simulink model "six_plus_six_AcmsteeringV09_main_2lfrf"  (R2014a)
settings: Solver=FixedStepDiscrete  StartTime=0.0  StopTime=10.0  FixedStep=0.0005  RelTol=1e-3
InitFcn:
  | Veh_Par_wxt
undefined symbols (not defined in the file or in its folder): acc_spdctl, ag_thr, B, bra_em, bra_pre_gz2, bra_pre_gz34, bra_pre_yd, brakepre_dem_data, brakeTrq_dem_data, bratrq_max, ecucoder_acal, eff_tran, ESP_switch, G, guzhang_lf, guzhang_lm, guzhang_lr, guzhang_rf, guzhang_rm, guzhang_rr, kd1, kd2, ki1, ki2, kp1, kp2, L, myFIS, premax, Radius, RC_switch, s_opt_yi, s_opt_zhuan, s_opt_zhuan_add, s_opt_zhuan_table, spd_map_mot, spd_spdctl, speed_thr_park, TCS_switch, tras_ratio, trq_map_mot, trqmax_yd, trqmax_zx, trqmaxneg, v_gain, v_table, v_thr_park, zhidong_bianmazhi, zhidong_down, zhidong_up, zhidong_youmen, zhuanxiang_bianmazhi, zhuanxiang_down, zhuanxiang_up, zhuanxiang_youmen
libraries: simulink x980, ec5744lib x59, fuzblock x2
(part 10 of 25)

== system six_plus_six_AcmsteeringV09_main_2lfrf/Data_input/MCU1_5/MCU1 ==
  input : Inport
  Enable : EnablePort
  Demux : Demux  Outputs=8
  MCU1_ControlTemp_Ad : Sum
  MCU1_ControlTemp_Convert : DataTypeConversion  OutDataTypeStr=uint32
  MCU1_ControlTemp_F : Gain
  MCU1_ControlTemp_L : simulink/Logic and Bit Operations/Bitwise Operator  logicop=AND  UseBitMask=on  BitMask=255  BitMaskRealWorld=Stored Integer
  MCU1_ControlTemp_O : Constant  Value=-40  OutDataTypeStr=single
  MCU1_ControlTemp_S : ArithShift
  MCU1_ControlTemp_Sub : Subsystem
  MCU1_ControlTemp_sat : Saturate  UpperLimit=215  LowerLimit=-40
  MCU1_ControlTempcv : DataTypeConversion
  MCU1_Idc_Ad : Sum
  MCU1_Idc_Convert : DataTypeConversion  OutDataTypeStr=uint32
  MCU1_Idc_F : Gain  Gain=0.1
  MCU1_Idc_L : simulink/Logic and Bit Operations/Bitwise Operator  logicop=AND  UseBitMask=on  BitMask=65535  BitMaskRealWorld=Stored Integer
  MCU1_Idc_O : Constant  Value=-1600  OutDataTypeStr=single
  MCU1_Idc_S : ArithShift
  MCU1_Idc_Sub : Subsystem
  MCU1_Idc_sat : Saturate  UpperLimit=1600  LowerLimit=-1600
  MCU1_Idccv : DataTypeConversion
  MCU1_Idcinput3_Ad : Sum
  MCU1_Idcinput3_C : Constant  Value=256
  MCU1_Idcinput3_P : Product
  MCU1_MotorTemp_Ad : Sum
  MCU1_MotorTemp_Convert : DataTypeConversion  OutDataTypeStr=uint32
  MCU1_MotorTemp_F : Gain
  MCU1_MotorTemp_L : simulink/Logic and Bit Operations/Bitwise Operator  logicop=AND  UseBitMask=on  BitMask=255  BitMaskRealWorld=Stored Integer
  MCU1_MotorTemp_O : Constant  Value=-40  OutDataTypeStr=single
  MCU1_MotorTemp_S : ArithShift
  MCU1_MotorTemp_Sub : Subsystem
  MCU1_MotorTemp_sat : Saturate  UpperLimit=215  LowerLimit=-40
  MCU1_MotorTempcv : DataTypeConversion
  MCU1_PowerFdk_Ad : Sum
  MCU1_PowerFdk_Convert : DataTypeConversion  OutDataTypeStr=uint32
  MCU1_PowerFdk_F : Gain
  MCU1_PowerFdk_L : simulink/Logic and Bit Operations/Bitwise Operator  logicop=AND  UseBitMask=on  BitMask=65535  BitMaskRealWorld=Stored Integer
  MCU1_PowerFdk_O : Constant  Value=0  OutDataTypeStr=single
  MCU1_PowerFdk_S : ArithShift
  MCU1_PowerFdk_Sub : Subsystem
  MCU1_PowerFdk_sat : Saturate  UpperLimit=65535  LowerLimit=0
  MCU1_PowerFdkcv : DataTypeConversion
  MCU1_PowerFdkinput5_Ad : Sum
  MCU1_PowerFdkinput5_C : Constant  Value=256
  MCU1_PowerFdkinput5_P : Product
  MCU1_Udc_Ad : Sum
  MCU1_Udc_Convert : DataTypeConversion  OutDataTypeStr=uint32
  MCU1_Udc_F : Gain  Gain=0.1
  MCU1_Udc_L : simulink/Logic and Bit Operations/Bitwise Operator  logicop=AND  UseBitMask=on  BitMask=65535  BitMaskRealWorld=Stored Integer
  MCU1_Udc_O : Constant  Value=0  OutDataTypeStr=single
  MCU1_Udc_S : ArithShift
  MCU1_Udc_Sub : Subsystem
  MCU1_Udc_sat : Saturate  UpperLimit=1000  LowerLimit=0
  MCU1_Udccv : DataTypeConversion
  MCU1_Udcinput1_Ad : Sum
  MCU1_Udcinput1_C : Constant  Value=256
  MCU1_Udcinput1_P : Product
  MCU1_ControlTemp_Out : Outport
  MCU1_MotorTemp_Out : Outport  Port=2
  MCU1_PowerFdk_Out : Outport  Port=3
  MCU1_Idc_Out : Outport  Port=4
  MCU1_Udc_Out : Outport  Port=5
  wires:
  MCU1_ControlTemp_F/1 -> MCU1_ControlTemp_Ad/1
  MCU1_ControlTemp_O/1 -> MCU1_ControlTemp_Ad/2
  MCU1_ControlTemp_Ad/1 -> MCU1_ControlTemp_sat/1
  MCU1_ControlTemp_sat/1 -> MCU1_ControlTemp_Out/1
  Demux/8 -> MCU1_ControlTemp_Sub/1(In1)
  MCU1_ControlTemp_Sub/1(Out1) -> MCU1_ControlTemp_Convert/1
  MCU1_ControlTemp_Convert/1 -> MCU1_ControlTemp_L/1
  MCU1_ControlTemp_L/1 -> MCU1_ControlTemp_S/1
  MCU1_ControlTemp_S/1 -> MCU1_ControlTempcv/1
  MCU1_ControlTempcv/1 -> MCU1_ControlTemp_F/1
  MCU1_MotorTemp_F/1 -> MCU1_MotorTemp_Ad/1
  MCU1_MotorTemp_O/1 -> MCU1_MotorTemp_Ad/2
  MCU1_MotorTemp_Ad/1 -> MCU1_MotorTemp_sat/1
  MCU1_MotorTemp_sat/1 -> MCU1_MotorTemp_Out/1
  Demux/7 -> MCU1_MotorTemp_Sub/1(In1)
  MCU1_MotorTemp_Sub/1(Out1) -> MCU1_MotorTemp_Convert/1
  MCU1_MotorTemp_Convert/1 -> MCU1_MotorTemp_L/1
  MCU1_MotorTemp_L/1 -> MCU1_MotorTemp_S/1
  MCU1_MotorTemp_S/1 -> MCU1_MotorTempcv/1
  MCU1_MotorTempcv/1 -> MCU1_MotorTemp_F/1
  MCU1_PowerFdk_F/1 -> MCU1_PowerFdk_Ad/1
  MCU1_PowerFdk_O/1 -> MCU1_PowerFdk_Ad/2
  MCU1_PowerFdk_Ad/1 -> MCU1_PowerFdk_sat/1
  MCU1_PowerFdk_sat/1 -> MCU1_PowerFdk_Out/1
  Demux/5 -> MCU1_PowerFdkinput5_P/1
  MCU1_PowerFdkinput5_C/1 -> MCU1_PowerFdkinput5_P/2
  MCU1_PowerFdkinput5_P/1 -> MCU1_PowerFdkinput5_Ad/1
  Demux/6 -> MCU1_PowerFdkinput5_Ad/2
  MCU1_PowerFdkinput5_Ad/1 -> MCU1_PowerFdk_Sub/1(In1)
  MCU1_PowerFdk_Sub/1(Out1) -> MCU1_PowerFdk_Convert/1
  MCU1_PowerFdk_Convert/1 -> MCU1_PowerFdk_L/1
  MCU1_PowerFdk_L/1 -> MCU1_PowerFdk_S/1
  MCU1_PowerFdk_S/1 -> MCU1_PowerFdkcv/1
  MCU1_PowerFdkcv/1 -> MCU1_PowerFdk_F/1
  MCU1_Idc_F/1 -> MCU1_Idc_Ad/1
  MCU1_Idc_O/1 -> MCU1_Idc_Ad/2
  MCU1_Idc_Ad/1 -> MCU1_Idc_sat/1
  MCU1_Idc_sat/1 -> MCU1_Idc_Out/1
  Demux/3 -> MCU1_Idcinput3_P/1
  MCU1_Idcinput3_C/1 -> MCU1_Idcinput3_P/2
  MCU1_Idcinput3_P/1 -> MCU1_Idcinput3_Ad/1
  Demux/4 -> MCU1_Idcinput3_Ad/2
  MCU1_Idcinput3_Ad/1 -> MCU1_Idc_Sub/1(In1)
  MCU1_Idc_Sub/1(Out1) -> MCU1_Idc_Convert/1
  MCU1_Idc_Convert/1 -> MCU1_Idc_L/1
  MCU1_Idc_L/1 -> MCU1_Idc_S/1
  MCU1_Idc_S/1 -> MCU1_Idccv/1
  MCU1_Idccv/1 -> MCU1_Idc_F/1
  MCU1_Udc_F/1 -> MCU1_Udc_Ad/1
  MCU1_Udc_O/1 -> MCU1_Udc_Ad/2
  MCU1_Udc_Ad/1 -> MCU1_Udc_sat/1
  MCU1_Udc_sat/1 -> MCU1_Udc_Out/1
  Demux/1 -> MCU1_Udcinput1_P/1
  MCU1_Udcinput1_C/1 -> MCU1_Udcinput1_P/2
  MCU1_Udcinput1_P/1 -> MCU1_Udcinput1_Ad/1
  Demux/2 -> MCU1_Udcinput1_Ad/2
  MCU1_Udcinput1_Ad/1 -> MCU1_Udc_Sub/1(In1)
  MCU1_Udc_Sub/1(Out1) -> MCU1_Udc_Convert/1
  MCU1_Udc_Convert/1 -> MCU1_Udc_L/1
  MCU1_Udc_L/1 -> MCU1_Udc_S/1
  MCU1_Udc_S/1 -> MCU1_Udccv/1
  MCU1_Udccv/1 -> MCU1_Udc_F/1
  input/1 -> Demux/1

== matlab function six_plus_six_AcmsteeringV09_main_2lfrf/MainControl/mode_control/backward/backward/Drive/目标转向力矩确定模块/MATLAB Function2 ==
  data: umax input; delta_Tsteer_max output; G input; L input; B input; Radius input; Rturn_min_xy input
function delta_Tsteer_max = fcn(umax,G,L,B,Radius,Rturn_min_xy)
%#codegen

    delta_Fsteer_max=single(umax/(0.925+0.15*(Rturn_min_xy/B))*G*L/(2*B));
    delta_Tsteer_max=single(delta_Fsteer_max*Radius);
    
end

== matlab function six_plus_six_AcmsteeringV09_main_2lfrf/MainControl/mode_control/backward/backward/Drive/驱动防滑控制TCS/直行TCS/直行/HeartBeat1 ==
  data: life_pre input; life output
function life = fcn(life_pre)
%#codegen
life=single(life_pre+1);
if life>255
    life=single(0);
end
end

== matlab function six_plus_six_AcmsteeringV09_main_2lfrf/MainControl/mode_control/backward/backward/Drive/驱动防滑控制TCS/直行TCS/直行/HeartBeat4 ==
  data: life_pre input; life output
function life = fcn(life_pre)
%#codegen
life=single(life_pre+1);
if life>255
    life=single(0);
end
end

== matlab function six_plus_six_AcmsteeringV09_main_2lfrf/MainControl/mode_control/forward/forward/Brake/Switch Case Action Subsystem/MATLAB Function5 ==
  data: bratrq_dem_lf input; bratrq_dem_lm input; bratrq_dem_lr input; bratrq_dem_rf input; bratrq_dem_rm input; bratrq_dem_rr input; pwr_chg_bat input; bratrq_mot_lf output; bratrq_mot_lm output; pwr_chg_bat1 input; pwr_chg_bat2 input; trqlimL_dig_lf input; bratrq_mot_lr output; bratrq_mot_rf output; bratrq_mot_rm output; bratrq_mot_rr output; trqlimL_dig_lm input; trqlimL_dig_lr input; trqlimL_dig_rf input; trqlimL_dig_rm input; trqlimL_dig_rr input; speed_act_lf input; speed_act_lm input; speed_act_lr input; speed_act_rf input; speed_act_rm input; speed_act_rr input; trqlim_map_lf input; brapre_out_l output; brapre_out_r output; trqlim_map_lm input; trqlim_map_lr input; trqlim_map_rf input; trqlim_map_rm input; trqlim_map_rr input; tras_ratio input; guzhang_lf input; guzhang_lm input; guzhang_lr input; guzhang_rf input; guzhang_rm input; guzhang_rr input
function [bratrq_mot_lf,bratrq_mot_lm,bratrq_mot_lr,bratrq_mot_rf,bratrq_mot_rm,bratrq_mot_rr,brapre_out_l,brapre_out_r] = fcn(bratrq_dem_lf,bratrq_dem_lm,bratrq_dem_lr,bratrq_dem_rf,bratrq_dem_rm,bratrq_dem_rr,pwr_chg_bat,pwr_chg_bat1,pwr_chg_bat2,trqlimL_dig_lf,trqlimL_dig_lm,trqlimL_dig_lr,trqlimL_dig_rf,trqlimL_dig_rm,trqlimL_dig_rr,speed_act_lf,speed_act_lm,speed_act_lr,speed_act_rf,speed_act_rm,speed_act_rr,trqlim_map_lf,trqlim_map_lm,trqlim_map_lr,trqlim_map_rf,trqlim_map_rm,trqlim_map_rr,tras_ratio,guzhang_lf,guzhang_lm,guzhang_lr,guzhang_rf,guzhang_rm,guzhang_rr)
%#codegen pid模块在外面做，里面进行十六种情况的判断，先看一下效果，不能再修改。前轴单独控制，后轴低选控制

bratrq_mot_lf1=single(bratrq_dem_lf/tras_ratio);
bratrq_mot_lf2=single(9549*(pwr_chg_bat/2)/speed_act_lf);
bratrq_mot_lf=single(min(trqlimL_dig_lf,min(bratrq_mot_lf1,bratrq_mot_lf2)));

bratrq_mot_lm1=single(bratrq_dem_lm/tras_ratio);
bratrq_mot_lm2=single(9549*(pwr_chg_bat1/2)/speed_act_lm);
bratrq_mot_lm=single(min(trqlimL_dig_lm,min(bratrq_mot_lm1,bratrq_mot_lm2)));

bratrq_mot_lr1=single(bratrq_dem_lr/tras_ratio);
bratrq_mot_lr2=single(9549*(pwr_chg_bat2/2)/speed_act_lr);
bratrq_mot_lr=single(min(trqlimL_dig_lr,min(bratrq_mot_lr1,bratrq_mot_lr2)));
 
bratrq_mot_rf1=single(bratrq_dem_rf/tras_ratio);
bratrq_mot_rf2=single(9549*(pwr_chg_bat/2)/speed_act_rf);
bratrq_mot_rf=single(min(trqlimL_dig_rf,min(bratrq_mot_rf1,bratrq_mot_rf2)));

bratrq_mot_rm1=single(bratrq_dem_rm/tras_ratio);
bratrq_mot_rm2=single(9549*(pwr_chg_bat1/2)/speed_act_rm);
bratrq_mot_rm=single(min(trqlimL_dig_rm,min(bratrq_mot_rm1,bratrq_mot_rm2)));

bratrq_mot_rr1=single(bratrq_dem_rr/tras_ratio);
bratrq_mot_rr2=single(9549*(pwr_chg_bat2/2)/speed_act_rr);
bratrq_mot_rr=single(min(trqlimL_dig_rr,min(bratrq_mot_rr1,bratrq_mot_rr2)));

brapre_out_l=single(((bratrq_dem_lf+bratrq_dem_lm+bratrq_dem_lr)-(bratrq_mot_lf+bratrq_mot_lm+bratrq_mot_lr)*tras_ratio)/3/150);
brapre_out_r=single(((bratrq_dem_rf+bratrq_dem_rm+bratrq_dem_rr)-(bratrq_mot_rf+bratrq_mot_rm+bratrq_mot_rr)*tras_ratio)/3/150);







bratrq_mot_lf=single(min(bratrq_mot_lf,trqlim_map_lf));%限一下最大值在外特性内，最小值大于0
bratrq_mot_lf=single(max(bratrq_mot_lf,0));
bratrq_mot_lr=single(min(bratrq_mot_lr,trqlim_map_lr));
bratrq_mot_lr=single(max(bratrq_mot_lr,0));
bratrq_mot_rf=single(min(bratrq_mot_rf,trqlim_map_rf));
bratrq_mot_rf=single(max(bratrq_mot_rf,0));
bratrq_mot_rr=single(min(bratrq_mot_rr,trqlim_map_rr));
bratrq_mot_rr=single(max(bratrq_mot_rr,0));

% brapre_out_l=brapre_out_l;
% brapre_out_r=brapre_out_r;
brapre_out_l=single(brapre_out_l*150/125);%第二辆车的制动压力与制动力的关系调整一下。
brapre_out_r=single(brapre_out_r*150/125);

if guzhang_lf==1
    bratrq_mot_lf=single(0);
end
if guzhang_lm==1
    bratrq_mot_lm=single(0);
end
if guzhang_lr==1
    bratrq_mot_lr=single(0);
end
if guzhang_rf==1
    bratrq_mot_rf=single(0);
end
if guzhang_rm==1
    bratrq_mot_rm=single(0);
end
if guzhang_rr==1
    bratrq_mot_rr=single(0);
end

end

== matlab function six_plus_six_AcmsteeringV09_main_2lfrf/MainControl/mode_control/Park/park/HeartBeat3 ==
  data: life_pre input; life output
function life = fcn(life_pre)
%#codegen
life=single(life_pre+1);
if life>255
    life=single(0);
end
end

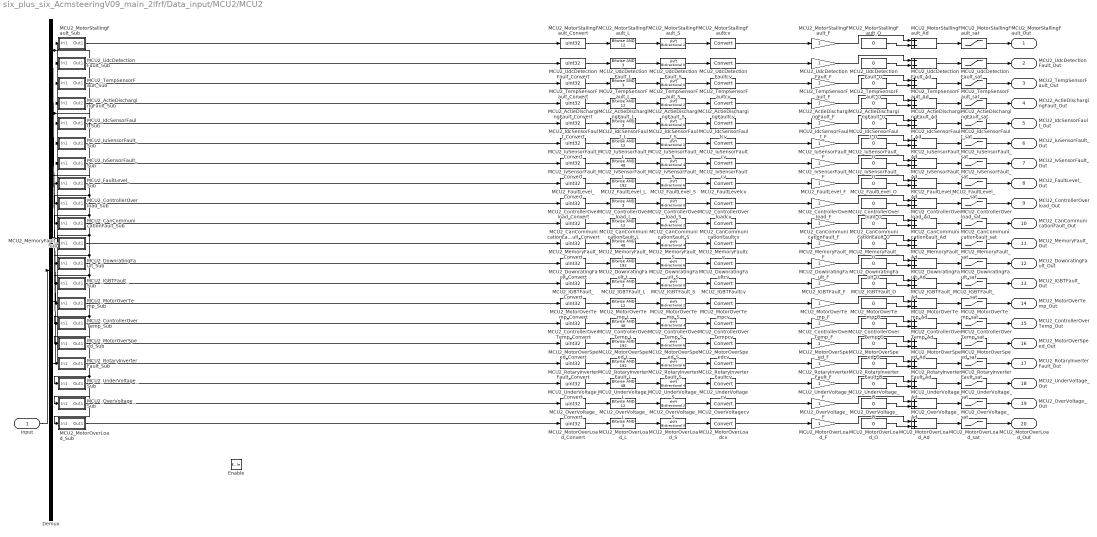
== system six_plus_six_AcmsteeringV09_main_2lfrf/Data_input/MCU2/MCU2 ==
  input : Inport
  Enable : EnablePort
  Demux : Demux  Outputs=8
  MCU2_ActieDischargingFault_Ad : Sum
  MCU2_ActieDischargingFault_Convert : DataTypeConversion  OutDataTypeStr=uint32
  MCU2_ActieDischargingFault_F : Gain
  MCU2_ActieDischargingFault_L : simulink/Logic and Bit Operations/Bitwise Operator  logicop=AND  UseBitMask=on  BitMask=12  BitMaskRealWorld=Stored Integer
  MCU2_ActieDischargingFault_O : Constant  Value=0  OutDataTypeStr=single
  MCU2_ActieDischargingFault_S : ArithShift  BitShiftNumber=2
  MCU2_ActieDischargingFault_Sub : Subsystem
  MCU2_ActieDischargingFault_sat : Saturate  UpperLimit=3  LowerLimit=0
  MCU2_ActieDischargingFaultcv : DataTypeConversion
  MCU2_CanCommunicationFault_Ad : Sum
  MCU2_CanCommunicationFault_Convert : DataTypeConversion  OutDataTypeStr=uint32
  MCU2_CanCommunicationFault_F : Gain
  MCU2_CanCommunicationFault_L : simulink/Logic and Bit Operations/Bitwise Operator  logicop=AND  UseBitMask=on  BitMask=12  BitMaskRealWorld=Stored Integer
  MCU2_CanCommunicationFault_O : Constant  Value=0  OutDataTypeStr=single
  MCU2_CanCommunicationFault_S : ArithShift  BitShiftNumber=2
  MCU2_CanCommunicationFault_Sub : Subsystem
  MCU2_CanCommunicationFault_sat : Saturate  UpperLimit=3  LowerLimit=0
  MCU2_CanCommunicationFaultcv : DataTypeConversion
  MCU2_ControllerOverTemp_Ad : Sum
  MCU2_ControllerOverTemp_Convert : DataTypeConversion  OutDataTypeStr=uint32
  MCU2_ControllerOverTemp_F : Gain
  MCU2_ControllerOverTemp_L : simulink/Logic and Bit Operations/Bitwise Operator  logicop=AND  UseBitMask=on  BitMask=48  BitMaskRealWorld=Stored Integer
  MCU2_ControllerOverTemp_O : Constant  Value=0  OutDataTypeStr=single
  MCU2_ControllerOverTemp_S : ArithShift  BitShiftNumber=4
  MCU2_ControllerOverTemp_Sub : Subsystem
  MCU2_ControllerOverTemp_sat : Saturate  UpperLimit=3  LowerLimit=0
  MCU2_ControllerOverTempcv : DataTypeConversion
  MCU2_ControllerOverload_Ad : Sum
  MCU2_ControllerOverload_Convert : DataTypeConversion  OutDataTypeStr=uint32
  MCU2_ControllerOverload_F : Gain
  MCU2_ControllerOverload_L : simulink/Logic and Bit Operations/Bitwise Operator  logicop=AND  UseBitMask=on  BitMask=3  BitMaskRealWorld=Stored Integer
  MCU2_ControllerOverload_O : Constant  Value=0  OutDataTypeStr=single
  MCU2_ControllerOverload_S : ArithShift
  MCU2_ControllerOverload_Sub : Subsystem
  MCU2_ControllerOverload_sat : Saturate  UpperLimit=3  LowerLimit=0
  MCU2_ControllerOverloadcv : DataTypeConversion
  MCU2_DownratingFault_Ad : Sum
  MCU2_DownratingFault_Convert : DataTypeConversion  OutDataTypeStr=uint32
  MCU2_DownratingFault_F : Gain
  MCU2_DownratingFault_L : simulink/Logic and Bit Operations/Bitwise Operator  logicop=AND  UseBitMask=on  BitMask=192  BitMaskRealWorld=Stored Integer
  MCU2_DownratingFault_O : Constant  Value=0  OutDataTypeStr=single
  MCU2_DownratingFault_S : ArithShift  BitShiftNumber=6
  MCU2_DownratingFault_Sub : Subsystem
  MCU2_DownratingFault_sat : Saturate  UpperLimit=3  LowerLimit=0
  MCU2_DownratingFaultcv : DataTypeConversion
  MCU2_FaultLevel_Ad : Sum
  MCU2_FaultLevel_Convert : DataTypeConversion  OutDataTypeStr=uint32
  MCU2_FaultLevel_F : Gain
  MCU2_FaultLevel_L : simulink/Logic and Bit Operations/Bitwise Operator  logicop=AND  UseBitMask=on  BitMask=192  BitMaskRealWorld=Stored Integer
  MCU2_FaultLevel_O : Constant  Value=0  OutDataTypeStr=single
  MCU2_FaultLevel_S : ArithShift  BitShiftNumber=6
  MCU2_FaultLevel_Sub : Subsystem
  MCU2_FaultLevel_sat : Saturate  UpperLimit=3  LowerLimit=0
  MCU2_FaultLevelcv : DataTypeConversion
  MCU2_IGBTFault_Ad : Sum
  MCU2_IGBTFault_Convert : DataTypeConversion  OutDataTypeStr=uint32
  MCU2_IGBTFault_F : Gain
  MCU2_IGBTFault_L : simulink/Logic and Bit Operations/Bitwise Operator  logicop=AND  UseBitMask=on  BitMask=3  BitMaskRealWorld=Stored Integer
  MCU2_IGBTFault_O : Constant  Value=0  OutDataTypeStr=single
  MCU2_IGBTFault_S : ArithShift
  MCU2_IGBTFault_Sub : Subsystem
  MCU2_IGBTFault_sat : Saturate  UpperLimit=3  LowerLimit=0
  MCU2_IGBTFaultcv : DataTypeConversion
  MCU2_IdcSensorFault_Ad : Sum
  MCU2_IdcSensorFault_Convert : DataTypeConversion  OutDataTypeStr=uint32
  MCU2_IdcSensorFault_F : Gain
  MCU2_IdcSensorFault_L : simulink/Logic and Bit Operations/Bitwise Operator  logicop=AND  UseBitMask=on  BitMask=3  BitMaskRealWorld=Stored Integer
  MCU2_IdcSensorFault_O : Constant  Value=0  OutDataTypeStr=single
  MCU2_IdcSensorFault_S : ArithShift
  MCU2_IdcSensorFault_Sub : Subsystem
  MCU2_IdcSensorFault_sat : Saturate  UpperLimit=3  LowerLimit=0
  MCU2_IdcSensorFaultcv : DataTypeConversion
  MCU2_IuSensorFault_Ad : Sum
  MCU2_IuSensorFault_Convert : DataTypeConversion  OutDataTypeStr=uint32
  MCU2_IuSensorFault_F : Gain
  MCU2_IuSensorFault_L : simulink/Logic and Bit Operations/Bitwise Operator  logicop=AND  UseBitMask=on  BitMask=12  BitMaskRealWorld=Stored Integer
  MCU2_IuSensorFault_O : Constant  Value=0  OutDataTypeStr=single
  MCU2_IuSensorFault_S : ArithShift  BitShiftNumber=2
  MCU2_IuSensorFault_Sub : Subsystem
  MCU2_IuSensorFault_sat : Saturate  UpperLimit=3  LowerLimit=0
  MCU2_IuSensorFaultcv : DataTypeConversion
  MCU2_IvSensorFault_Ad : Sum
  MCU2_IvSensorFault_Convert : DataTypeConversion  OutDataTypeStr=uint32
  MCU2_IvSensorFault_F : Gain
  MCU2_IvSensorFault_L : simulink/Logic and Bit Operations/Bitwise Operator  logicop=AND  UseBitMask=on  BitMask=48  BitMaskRealWorld=Stored Integer
  MCU2_IvSensorFault_O : Constant  Value=0  OutDataTypeStr=single
  MCU2_IvSensorFault_S : ArithShift  BitShiftNumber=4
  MCU2_IvSensorFault_Sub : Subsystem
  MCU2_IvSensorFault_sat : Saturate  UpperLimit=3  LowerLimit=0
  MCU2_IvSensorFaultcv : DataTypeConversion
  MCU2_MemoryFault_Ad : Sum
  MCU2_MemoryFault_Convert : DataTypeConversion  OutDataTypeStr=uint32
  MCU2_MemoryFault_F : Gain
  MCU2_MemoryFault_L : simulink/Logic and Bit Operations/Bitwise Operator  logicop=AND  UseBitMask=on  BitMask=48  BitMaskRealWorld=Stored Integer
  MCU2_MemoryFault_O : Constant  Value=0  OutDataTypeStr=single
  MCU2_MemoryFault_S : ArithShift  BitShiftNumber=4
  MCU2_MemoryFault_Sub : Subsystem
  MCU2_MemoryFault_sat : Saturate  UpperLimit=3  LowerLimit=0
  MCU2_MemoryFaultcv : DataTypeConversion
  MCU2_MotorOverLoad_Ad : Sum
  MCU2_MotorOverLoad_Convert : DataTypeConversion  OutDataTypeStr=uint32
  MCU2_MotorOverLoad_F : Gain
  MCU2_MotorOverLoad_L : simulink/Logic and Bit Operations/Bitwise Operator  logicop=AND  UseBitMask=on  BitMask=3  BitMaskRealWorld=Stored Integer
  MCU2_MotorOverLoad_O : Constant  Value=0  OutDataTypeStr=single
  MCU2_MotorOverLoad_S : ArithShift
  MCU2_MotorOverLoad_Sub : Subsystem
  MCU2_MotorOverLoad_sat : Saturate  UpperLimit=3  LowerLimit=0
  MCU2_MotorOverLoadcv : DataTypeConversion
  MCU2_MotorOverSpeed_Ad : Sum
  MCU2_MotorOverSpeed_Convert : DataTypeConversion  OutDataTypeStr=uint32
  MCU2_MotorOverSpeed_F : Gain
  MCU2_MotorOverSpeed_L : simulink/Logic and Bit Operations/Bitwise Operator  logicop=AND  UseBitMask=on  BitMask=192  BitMaskRealWorld=Stored Integer
  MCU2_MotorOverSpeed_O : Constant  Value=0  OutDataTypeStr=single
  MCU2_MotorOverSpeed_S : ArithShift  BitShiftNumber=6
  MCU2_MotorOverSpeed_Sub : Subsystem
  MCU2_MotorOverSpeed_sat : Saturate  UpperLimit=3  LowerLimit=0
  MCU2_MotorOverSpeedcv : DataTypeConversion
  MCU2_MotorOverTemp_Ad : Sum
  MCU2_MotorOverTemp_Convert : DataTypeConversion  OutDataTypeStr=uint32
  MCU2_MotorOverTemp_F : Gain
  MCU2_MotorOverTemp_L : simulink/Logic and Bit Operations/Bitwise Operator  logicop=AND  UseBitMask=on  BitMask=12  BitMaskRealWorld=Stored Integer
  MCU2_MotorOverTemp_O : Constant  Value=0  OutDataTypeStr=single
  MCU2_MotorOverTemp_S : ArithShift  BitShiftNumber=2
  MCU2_MotorOverTemp_Sub : Subsystem
  MCU2_MotorOverTemp_sat : Saturate  UpperLimit=3  LowerLimit=0
  MCU2_MotorOverTempcv : DataTypeConversion
  MCU2_MotorStallingFault_Ad : Sum
  MCU2_MotorStallingFault_Convert : DataTypeConversion  OutDataTypeStr=uint32
  MCU2_MotorStallingFault_F : Gain
  MCU2_MotorStallingFault_L : simulink/Logic and Bit Operations/Bitwise Operator  logicop=AND  UseBitMask=on  BitMask=12  BitMaskRealWorld=Stored Integer
  MCU2_MotorStallingFault_O : Constant  Value=0  OutDataTypeStr=single
  MCU2_MotorStallingFault_S : ArithShift  BitShiftNumber=2
  MCU2_MotorStallingFault_Sub : Subsystem
  MCU2_MotorStallingFault_sat : Saturate  UpperLimit=3  LowerLimit=0
  MCU2_MotorStallingFaultcv : DataTypeConversion
  MCU2_OverVoltage_Ad : Sum
  MCU2_OverVoltage_Convert : DataTypeConversion  OutDataTypeStr=uint32
  MCU2_OverVoltage_F : Gain
  MCU2_OverVoltage_L : simulink/Logic and Bit Operations/Bitwise Operator  logicop=AND  UseBitMask=on  BitMask=12  BitMaskRealWorld=Stored Integer
  MCU2_OverVoltage_O : Constant  Value=0  OutDataTypeStr=single
  MCU2_OverVoltage_S : ArithShift  BitShiftNumber=2
  MCU2_OverVoltage_Sub : Subsystem
  MCU2_OverVoltage_sat : Saturate  UpperLimit=3  LowerLimit=0
  MCU2_OverVoltagecv : DataTypeConversion
  MCU2_RotaryInverterFault_Ad : Sum
  MCU2_RotaryInverterFault_Convert : DataTypeConversion  OutDataTypeStr=uint32
  MCU2_RotaryInverterFault_F : Gain
  MCU2_RotaryInverterFault_L : simulink/Logic and Bit Operations/Bitwise Operator  logicop=AND  UseBitMask=on  BitMask=192  BitMaskRealWorld=Stored Integer
  MCU2_RotaryInverterFault_O : Constant  Value=0  OutDataTypeStr=single
  MCU2_RotaryInverterFault_S : ArithShift  BitShiftNumber=6
  MCU2_RotaryInverterFault_Sub : Subsystem
  MCU2_RotaryInverterFault_sat : Saturate  UpperLimit=3  LowerLimit=0
  MCU2_RotaryInverterFaultcv : DataTypeConversion
  MCU2_TempSensorFault_Ad : Sum
  MCU2_TempSensorFault_Convert : DataTypeConversion  OutDataTypeStr=uint32
  MCU2_TempSensorFault_F : Gain
  MCU2_TempSensorFault_L : simulink/Logic and Bit Operations/Bitwise Operator  logicop=AND  UseBitMask=on  BitMask=3  BitMaskRealWorld=Stored Integer
  MCU2_TempSensorFault_O : Constant  Value=0  OutDataTypeStr=single
  MCU2_TempSensorFault_S : ArithShift
  MCU2_TempSensorFault_Sub : Subsystem
  MCU2_TempSensorFault_sat : Saturate  UpperLimit=3  LowerLimit=0
  MCU2_TempSensorFaultcv : DataTypeConversion
  MCU2_UdcDetectionFault_Ad : Sum
  MCU2_UdcDetectionFault_Convert : DataTypeConversion  OutDataTypeStr=uint32
  MCU2_UdcDetectionFault_F : Gain
  MCU2_UdcDetectionFault_L : simulink/Logic and Bit Operations/Bitwise Operator  logicop=AND  UseBitMask=on  BitMask=3  BitMaskRealWorld=Stored Integer
  MCU2_UdcDetectionFault_O : Constant  Value=0  OutDataTypeStr=single
  MCU2_UdcDetectionFault_S : ArithShift
  MCU2_UdcDetectionFault_Sub : Subsystem
  MCU2_UdcDetectionFault_sat : Saturate  UpperLimit=3  LowerLimit=0
  MCU2_UdcDetectionFaultcv : DataTypeConversion
  MCU2_UnderVoltage_Ad : Sum
  MCU2_UnderVoltage_Convert : DataTypeConversion  OutDataTypeStr=uint32
  MCU2_UnderVoltage_F : Gain
  MCU2_UnderVoltage_L : simulink/Logic and Bit Operations/Bitwise Operator  logicop=AND  UseBitMask=on  BitMask=48  BitMaskRealWorld=Stored Integer
  MCU2_UnderVoltage_O : Constant  Value=0  OutDataTypeStr=single
  MCU2_UnderVoltage_S : ArithShift  BitShiftNumber=4
  MCU2_UnderVoltage_Sub : Subsystem
  MCU2_UnderVoltage_sat : Saturate  UpperLimit=3  LowerLimit=0
  MCU2_UnderVoltagecv : DataTypeConversion
  MCU2_MotorStallingFault_Out : Outport
  MCU2_UdcDetectionFault_Out : Outport  Port=2
  MCU2_TempSensorFault_Out : Outport  Port=3
  MCU2_ActieDischargingFault_Out : Outport  Port=4
  MCU2_IdcSensorFault_Out : Outport  Port=5
  MCU2_IuSensorFault_Out : Outport  Port=6
  MCU2_IvSensorFault_Out : Outport  Port=7
  MCU2_FaultLevel_Out : Outport  Port=8
  MCU2_ControllerOverload_Out : Outport  Port=9
  MCU2_CanCommunicationFault_Out : Outport  Port=10
  MCU2_MemoryFault_Out : Outport  Port=11
  MCU2_DownratingFault_Out : Outport  Port=12
  MCU2_IGBTFault_Out : Outport  Port=13
  MCU2_MotorOverTemp_Out : Outport  Port=14
  MCU2_ControllerOverTemp_Out : Outport  Port=15
  MCU2_MotorOverSpeed_Out : Outport  Port=16
  MCU2_RotaryInverterFault_Out : Outport  Port=17
  MCU2_UnderVoltage_Out : Outport  Port=18
  MCU2_OverVoltage_Out : Outport  Port=19
  MCU2_MotorOverLoad_Out : Outport  Port=20
  wires:
  MCU2_MotorStallingFault_F/1 -> MCU2_MotorStallingFault_Ad/1
  MCU2_MotorStallingFault_O/1 -> MCU2_MotorStallingFault_Ad/2
  MCU2_MotorStallingFault_Ad/1 -> MCU2_MotorStallingFault_sat/1
  MCU2_MotorStallingFault_sat/1 -> MCU2_MotorStallingFault_Out/1
  Demux/6 -> MCU2_MotorStallingFault_Sub/1(In1), MCU2_UdcDetectionFault_Sub/1(In1)
  MCU2_MotorStallingFault_Sub/1(Out1) -> MCU2_MotorStallingFault_Convert/1
  MCU2_MotorStallingFault_Convert/1 -> MCU2_MotorStallingFault_L/1
  MCU2_MotorStallingFault_L/1 -> MCU2_MotorStallingFault_S/1
  MCU2_MotorStallingFault_S/1 -> MCU2_MotorStallingFaultcv/1
  MCU2_MotorStallingFaultcv/1 -> MCU2_MotorStallingFault_F/1
  MCU2_UdcDetectionFault_F/1 -> MCU2_UdcDetectionFault_Ad/1
  MCU2_UdcDetectionFault_O/1 -> MCU2_UdcDetectionFault_Ad/2
  MCU2_UdcDetectionFault_Ad/1 -> MCU2_UdcDetectionFault_sat/1
  MCU2_UdcDetectionFault_sat/1 -> MCU2_UdcDetectionFault_Out/1
  MCU2_UdcDetectionFault_Sub/1(Out1) -> MCU2_UdcDetectionFault_Convert/1
  MCU2_UdcDetectionFault_Convert/1 -> MCU2_UdcDetectionFault_L/1
  MCU2_UdcDetectionFault_L/1 -> MCU2_UdcDetectionFault_S/1
  MCU2_UdcDetectionFault_S/1 -> MCU2_UdcDetectionFaultcv/1
  MCU2_UdcDetectionFaultcv/1 -> MCU2_UdcDetectionFault_F/1
  MCU2_TempSensorFault_F/1 -> MCU2_TempSensorFault_Ad/1
  MCU2_TempSensorFault_O/1 -> MCU2_TempSensorFault_Ad/2
  MCU2_TempSensorFault_Ad/1 -> MCU2_TempSensorFault_sat/1
  MCU2_TempSensorFault_sat/1 -> MCU2_TempSensorFault_Out/1
  Demux/5 -> MCU2_TempSensorFault_Sub/1(In1), MCU2_ActieDischargingFault_Sub/1(In1)
  MCU2_TempSensorFault_Sub/1(Out1) -> MCU2_TempSensorFault_Convert/1
  MCU2_TempSensorFault_Convert/1 -> MCU2_TempSensorFault_L/1
  MCU2_TempSensorFault_L/1 -> MCU2_TempSensorFault_S/1
  MCU2_TempSensorFault_S/1 -> MCU2_TempSensorFaultcv/1
  MCU2_TempSensorFaultcv/1 -> MCU2_TempSensorFault_F/1
  MCU2_ActieDischargingFault_F/1 -> MCU2_ActieDischargingFault_Ad/1
  MCU2_ActieDischargingFault_O/1 -> MCU2_ActieDischargingFault_Ad/2
  MCU2_ActieDischargingFault_Ad/1 -> MCU2_ActieDischargingFault_sat/1
  MCU2_ActieDischargingFault_sat/1 -> MCU2_ActieDischargingFault_Out/1
  MCU2_ActieDischargingFault_Sub/1(Out1) -> MCU2_ActieDischargingFault_Convert/1
  MCU2_ActieDischargingFault_Convert/1 -> MCU2_ActieDischargingFault_L/1
  MCU2_ActieDischargingFault_L/1 -> MCU2_ActieDischargingFault_S/1
  MCU2_ActieDischargingFault_S/1 -> MCU2_ActieDischargingFaultcv/1
  MCU2_ActieDischargingFaultcv/1 -> MCU2_ActieDischargingFault_F/1
  MCU2_IdcSensorFault_F/1 -> MCU2_IdcSensorFault_Ad/1
  MCU2_IdcSensorFault_O/1 -> MCU2_IdcSensorFault_Ad/2
  MCU2_IdcSensorFault_Ad/1 -> MCU2_IdcSensorFault_sat/1
  MCU2_IdcSensorFault_sat/1 -> MCU2_IdcSensorFault_Out/1
  Demux/4 -> MCU2_IdcSensorFault_Sub/1(In1), MCU2_IuSensorFault_Sub/1(In1), MCU2_IvSensorFault_Sub/1(In1), MCU2_FaultLevel_Sub/1(In1)
  MCU2_IdcSensorFault_Sub/1(Out1) -> MCU2_IdcSensorFault_Convert/1
  MCU2_IdcSensorFault_Convert/1 -> MCU2_IdcSensorFault_L/1
  MCU2_IdcSensorFault_L/1 -> MCU2_IdcSensorFault_S/1
  MCU2_IdcSensorFault_S/1 -> MCU2_IdcSensorFaultcv/1
  MCU2_IdcSensorFaultcv/1 -> MCU2_IdcSensorFault_F/1
  MCU2_IuSensorFault_F/1 -> MCU2_IuSensorFault_Ad/1
  MCU2_IuSensorFault_O/1 -> MCU2_IuSensorFault_Ad/2
  MCU2_IuSensorFault_Ad/1 -> MCU2_IuSensorFault_sat/1
  MCU2_IuSensorFault_sat/1 -> MCU2_IuSensorFault_Out/1
  MCU2_IuSensorFault_Sub/1(Out1) -> MCU2_IuSensorFault_Convert/1
  MCU2_IuSensorFault_Convert/1 -> MCU2_IuSensorFault_L/1
  MCU2_IuSensorFault_L/1 -> MCU2_IuSensorFault_S/1
  MCU2_IuSensorFault_S/1 -> MCU2_IuSensorFaultcv/1
  MCU2_IuSensorFaultcv/1 -> MCU2_IuSensorFault_F/1
  MCU2_IvSensorFault_F/1 -> MCU2_IvSensorFault_Ad/1
  MCU2_IvSensorFault_O/1 -> MCU2_IvSensorFault_Ad/2
  MCU2_IvSensorFault_Ad/1 -> MCU2_IvSensorFault_sat/1
  MCU2_IvSensorFault_sat/1 -> MCU2_IvSensorFault_Out/1
  MCU2_IvSensorFault_Sub/1(Out1) -> MCU2_IvSensorFault_Convert/1
  MCU2_IvSensorFault_Convert/1 -> MCU2_IvSensorFault_L/1
  MCU2_IvSensorFault_L/1 -> MCU2_IvSensorFault_S/1
  MCU2_IvSensorFault_S/1 -> MCU2_IvSensorFaultcv/1
  MCU2_IvSensorFaultcv/1 -> MCU2_IvSensorFault_F/1
  MCU2_FaultLevel_F/1 -> MCU2_FaultLevel_Ad/1
  MCU2_FaultLevel_O/1 -> MCU2_FaultLevel_Ad/2
  MCU2_FaultLevel_Ad/1 -> MCU2_FaultLevel_sat/1
  MCU2_FaultLevel_sat/1 -> MCU2_FaultLevel_Out/1
  MCU2_FaultLevel_Sub/1(Out1) -> MCU2_FaultLevel_Convert/1
  MCU2_FaultLevel_Convert/1 -> MCU2_FaultLevel_L/1
  MCU2_FaultLevel_L/1 -> MCU2_FaultLevel_S/1
  MCU2_FaultLevel_S/1 -> MCU2_FaultLevelcv/1
  MCU2_FaultLevelcv/1 -> MCU2_FaultLevel_F/1
  MCU2_ControllerOverload_F/1 -> MCU2_ControllerOverload_Ad/1
  MCU2_ControllerOverload_O/1 -> MCU2_ControllerOverload_Ad/2
  MCU2_ControllerOverload_Ad/1 -> MCU2_ControllerOverload_sat/1
  MCU2_ControllerOverload_sat/1 -> MCU2_ControllerOverload_Out/1
  Demux/1 -> MCU2_UnderVoltage_Sub/1(In1), MCU2_OverVoltage_Sub/1(In1), MCU2_ControllerOverload_Sub/1(In1), MCU2_RotaryInverterFault_Sub/1(In1)
  MCU2_ControllerOverload_Sub/1(Out1) -> MCU2_ControllerOverload_Convert/1
  MCU2_ControllerOverload_Convert/1 -> MCU2_ControllerOverload_L/1
  MCU2_ControllerOverload_L/1 -> MCU2_ControllerOverload_S/1
  MCU2_ControllerOverload_S/1 -> MCU2_ControllerOverloadcv/1
  MCU2_ControllerOverloadcv/1 -> MCU2_ControllerOverload_F/1
  MCU2_CanCommunicationFault_F/1 -> MCU2_CanCommunicationFault_Ad/1
  MCU2_CanCommunicationFault_O/1 -> MCU2_CanCommunicationFault_Ad/2
  MCU2_CanCommunicationFault_Ad/1 -> MCU2_CanCommunicationFault_sat/1
  MCU2_CanCommunicationFault_sat/1 -> MCU2_CanCommunicationFault_Out/1
  Demux/3 -> MCU2_DownratingFault_Sub/1(In1), MCU2_MotorOverLoad_Sub/1(In1), MCU2_MemoryFault_Sub/1(In1), MCU2_CanCommunicationFault_Sub/1(In1)
  MCU2_CanCommunicationFault_Sub/1(Out1) -> MCU2_CanCommunicationFault_Convert/1
  MCU2_CanCommunicationFault_Convert/1 -> MCU2_CanCommunicationFault_L/1
  MCU2_CanCommunicationFault_L/1 -> MCU2_CanCommunicationFault_S/1
  MCU2_CanCommunicationFault_S/1 -> MCU2_CanCommunicationFaultcv/1
  MCU2_CanCommunicationFaultcv/1 -> MCU2_CanCommunicationFault_F/1
  MCU2_MemoryFault_F/1 -> MCU2_MemoryFault_Ad/1
  MCU2_MemoryFault_O/1 -> MCU2_MemoryFault_Ad/2
  MCU2_MemoryFault_Ad/1 -> MCU2_MemoryFault_sat/1
  MCU2_MemoryFault_sat/1 -> MCU2_MemoryFault_Out/1
  MCU2_MemoryFault_Sub/1(Out1) -> MCU2_MemoryFault_Convert/1
  MCU2_MemoryFault_Convert/1 -> MCU2_MemoryFault_L/1
  MCU2_MemoryFault_L/1 -> MCU2_MemoryFault_S/1
  MCU2_MemoryFault_S/1 -> MCU2_MemoryFaultcv/1
  MCU2_MemoryFaultcv/1 -> MCU2_MemoryFault_F/1
  MCU2_DownratingFault_F/1 -> MCU2_DownratingFault_Ad/1
  MCU2_DownratingFault_O/1 -> MCU2_DownratingFault_Ad/2
  MCU2_DownratingFault_Ad/1 -> MCU2_DownratingFault_sat/1
  MCU2_DownratingFault_sat/1 -> MCU2_DownratingFault_Out/1
  MCU2_DownratingFault_Sub/1(Out1) -> MCU2_DownratingFault_Convert/1
  MCU2_DownratingFault_Convert/1 -> MCU2_DownratingFault_L/1
  MCU2_DownratingFault_L/1 -> MCU2_DownratingFault_S/1
  MCU2_DownratingFault_S/1 -> MCU2_DownratingFaultcv/1
  MCU2_DownratingFaultcv/1 -> MCU2_DownratingFault_F/1
  MCU2_IGBTFault_F/1 -> MCU2_IGBTFault_Ad/1
  MCU2_IGBTFault_O/1 -> MCU2_IGBTFault_Ad/2
  MCU2_IGBTFault_Ad/1 -> MCU2_IGBTFault_sat/1
  MCU2_IGBTFault_sat/1 -> MCU2_IGBTFault_Out/1
  Demux/2 -> MCU2_ControllerOverTemp_Sub/1(In1), MCU2_MotorOverSpeed_Sub/1(In1), MCU2_IGBTFault_Sub/1(In1), MCU2_MotorOverTemp_Sub/1(In1)
  MCU2_IGBTFault_Sub/1(Out1) -> MCU2_IGBTFault_Convert/1
  MCU2_IGBTFault_Convert/1 -> MCU2_IGBTFault_L/1
  MCU2_IGBTFault_L/1 -> MCU2_IGBTFault_S/1
  MCU2_IGBTFault_S/1 -> MCU2_IGBTFaultcv/1
  MCU2_IGBTFaultcv/1 -> MCU2_IGBTFault_F/1
  MCU2_MotorOverTemp_F/1 -> MCU2_MotorOverTemp_Ad/1
  MCU2_MotorOverTemp_O/1 -> MCU2_MotorOverTemp_Ad/2
  MCU2_MotorOverTemp_Ad/1 -> MCU2_MotorOverTemp_sat/1
  MCU2_MotorOverTemp_sat/1 -> MCU2_MotorOverTemp_Out/1
  MCU2_MotorOverTemp_Sub/1(Out1) -> MCU2_MotorOverTemp_Convert/1
  MCU2_MotorOverTemp_Convert/1 -> MCU2_MotorOverTemp_L/1
  MCU2_MotorOverTemp_L/1 -> MCU2_MotorOverTemp_S/1
  MCU2_MotorOverTemp_S/1 -> MCU2_MotorOverTempcv/1
  MCU2_MotorOverTempcv/1 -> MCU2_MotorOverTemp_F/1
  MCU2_ControllerOverTemp_F/1 -> MCU2_ControllerOverTemp_Ad/1
  MCU2_ControllerOverTemp_O/1 -> MCU2_ControllerOverTemp_Ad/2
  MCU2_ControllerOverTemp_Ad/1 -> MCU2_ControllerOverTemp_sat/1
  MCU2_ControllerOverTemp_sat/1 -> MCU2_ControllerOverTemp_Out/1
  MCU2_ControllerOverTemp_Sub/1(Out1) -> MCU2_ControllerOverTemp_Convert/1
  MCU2_ControllerOverTemp_Convert/1 -> MCU2_ControllerOverTemp_L/1
  MCU2_ControllerOverTemp_L/1 -> MCU2_ControllerOverTemp_S/1
  MCU2_ControllerOverTemp_S/1 -> MCU2_ControllerOverTempcv/1
  MCU2_ControllerOverTempcv/1 -> MCU2_ControllerOverTemp_F/1
  MCU2_MotorOverSpeed_F/1 -> MCU2_MotorOverSpeed_Ad/1
  MCU2_MotorOverSpeed_O/1 -> MCU2_MotorOverSpeed_Ad/2
  MCU2_MotorOverSpeed_Ad/1 -> MCU2_MotorOverSpeed_sat/1
  MCU2_MotorOverSpeed_sat/1 -> MCU2_MotorOverSpeed_Out/1
  MCU2_MotorOverSpeed_Sub/1(Out1) -> MCU2_MotorOverSpeed_Convert/1
  MCU2_MotorOverSpeed_Convert/1 -> MCU2_MotorOverSpeed_L/1
  MCU2_MotorOverSpeed_L/1 -> MCU2_MotorOverSpeed_S/1
  MCU2_MotorOverSpeed_S/1 -> MCU2_MotorOverSpeedcv/1
  MCU2_MotorOverSpeedcv/1 -> MCU2_MotorOverSpeed_F/1
  MCU2_RotaryInverterFault_F/1 -> MCU2_RotaryInverterFault_Ad/1
  MCU2_RotaryInverterFault_O/1 -> MCU2_RotaryInverterFault_Ad/2
  MCU2_RotaryInverterFault_Ad/1 -> MCU2_RotaryInverterFault_sat/1
  MCU2_RotaryInverterFault_sat/1 -> MCU2_RotaryInverterFault_Out/1
  MCU2_RotaryInverterFault_Sub/1(Out1) -> MCU2_RotaryInverterFault_Convert/1
  MCU2_RotaryInverterFault_Convert/1 -> MCU2_RotaryInverterFault_L/1
  MCU2_RotaryInverterFault_L/1 -> MCU2_RotaryInverterFault_S/1
  MCU2_RotaryInverterFault_S/1 -> MCU2_RotaryInverterFaultcv/1
  MCU2_RotaryInverterFaultcv/1 -> MCU2_RotaryInverterFault_F/1
  MCU2_UnderVoltage_F/1 -> MCU2_UnderVoltage_Ad/1
  MCU2_UnderVoltage_O/1 -> MCU2_UnderVoltage_Ad/2
  MCU2_UnderVoltage_Ad/1 -> MCU2_UnderVoltage_sat/1
  MCU2_UnderVoltage_sat/1 -> MCU2_UnderVoltage_Out/1
  MCU2_UnderVoltage_Sub/1(Out1) -> MCU2_UnderVoltage_Convert/1
  MCU2_UnderVoltage_Convert/1 -> MCU2_UnderVoltage_L/1
  MCU2_UnderVoltage_L/1 -> MCU2_UnderVoltage_S/1
  MCU2_UnderVoltage_S/1 -> MCU2_UnderVoltagecv/1
  MCU2_UnderVoltagecv/1 -> MCU2_UnderVoltage_F/1
  MCU2_OverVoltage_F/1 -> MCU2_OverVoltage_Ad/1
  MCU2_OverVoltage_O/1 -> MCU2_OverVoltage_Ad/2
  MCU2_OverVoltage_Ad/1 -> MCU2_OverVoltage_sat/1
  MCU2_OverVoltage_sat/1 -> MCU2_OverVoltage_Out/1
  MCU2_OverVoltage_Sub/1(Out1) -> MCU2_OverVoltage_Convert/1
  MCU2_OverVoltage_Convert/1 -> MCU2_OverVoltage_L/1
  MCU2_OverVoltage_L/1 -> MCU2_OverVoltage_S/1
  MCU2_OverVoltage_S/1 -> MCU2_OverVoltagecv/1
  MCU2_OverVoltagecv/1 -> MCU2_OverVoltage_F/1
  MCU2_MotorOverLoad_F/1 -> MCU2_MotorOverLoad_Ad/1
  MCU2_MotorOverLoad_O/1 -> MCU2_MotorOverLoad_Ad/2
  MCU2_MotorOverLoad_Ad/1 -> MCU2_MotorOverLoad_sat/1
  MCU2_MotorOverLoad_sat/1 -> MCU2_MotorOverLoad_Out/1
  MCU2_MotorOverLoad_Sub/1(Out1) -> MCU2_MotorOverLoad_Convert/1
  MCU2_MotorOverLoad_Convert/1 -> MCU2_MotorOverLoad_L/1
  MCU2_MotorOverLoad_L/1 -> MCU2_MotorOverLoad_S/1
  MCU2_MotorOverLoad_S/1 -> MCU2_MotorOverLoadcv/1
  MCU2_MotorOverLoadcv/1 -> MCU2_MotorOverLoad_F/1
  input/1 -> Demux/1
